simulink model "sis_cascata_discreto"  (R2019b)
settings: Solver=VariableStepAuto  StartTime=0.0  StopTime=10.0  RelTol=1e-3
undefined symbols (not defined in the file or in its folder): den_G1, den_G2, den_Raa_i, den_Raa_o, den_Rpf, DENdi, DENdo, num_G1, num_G2, num_Raa_i, num_Raa_o, num_Rpf, NUMdi, NUMdo, Ts_i, Ts_o
settings Model: Creator=edoardo  LastModifiedBy=edoardo

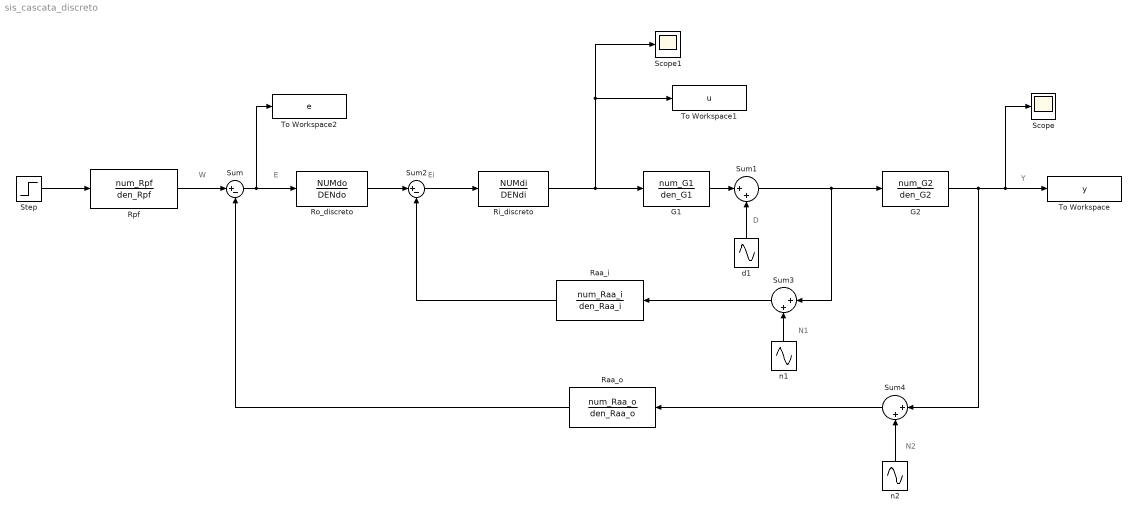
== system sis_cascata_discreto ==
  note: W
  note: Y
  note: Ei
  note: E
  note: D
  note: N1
  note: N2
  "G1 " : TransferFcn  Numerator=num_G1  Denominator=den_G1
  G2 : TransferFcn  Numerator=num_G2  Denominator=den_G2
  Raa_i : TransferFcn  Numerator=num_Raa_i  Denominator=den_Raa_i
  Raa_o : TransferFcn  Numerator=num_Raa_o  Denominator=den_Raa_o
  "Ri_discreto " : DiscreteTransferFcn  Numerator=NUMdi  Denominator=DENdi  SampleTime=Ts_i
  "Ro_discreto " : DiscreteTransferFcn  Numerator=NUMdo  Denominator=DENdo  SampleTime=Ts_o
  "Rpf " : TransferFcn  Numerator=num_Rpf  Denominator=den_Rpf
  Scope : Scope
  Scope1 : Scope
  Step : Step  Time=0  After=1.5  SampleTime=0
  Sum : Sum  Inputs=|+-
  Sum1 : Sum  Inputs=|++
  Sum2 : Sum  Inputs=|+-
  Sum3 : Sum  Inputs=|++
  Sum4 : Sum  Inputs=|++
  To Workspace : ToWorkspace  VariableName=y  SaveFormat=Timeseries  SampleTime=-1
  To Workspace1 : ToWorkspace  VariableName=u  SaveFormat=Timeseries  SampleTime=-1
  To Workspace2 : ToWorkspace  VariableName=e  SaveFormat=Timeseries  SampleTime=-1
  d1 : Sin  Amplitude=3  SampleTime=0
  n1 : Sin  Amplitude=0.02  Frequency=8000  SampleTime=0
  n2 : Sin  Amplitude=0.02  Frequency=8000  SampleTime=0
  wires:
  Sum/1 -> "Ro_discreto "/1, To Workspace2/1
  Sum1/1 -> Sum3/1, G2/1
  Sum2/1 -> "Ri_discreto "/1
  n2/1 -> Sum4/2
  "Rpf "/1 -> Sum/1
  "Ri_discreto "/1 -> To Workspace1/1, Scope1/1, "G1 "/1
  G2/1 -> Sum4/1, Scope/1, To Workspace/1
  d1/1 -> Sum1/2
  "Ro_discreto "/1 -> Sum2/1
  "G1 "/1 -> Sum1/1
  Step/1 -> "Rpf "/1
  n1/1 -> Sum3/2
  Sum3/1 -> Raa_i/1
  Raa_i/1 -> Sum2/2
  Sum4/1 -> Raa_o/1
  Raa_o/1 -> Sum/2
